simulink model "pendule_simple"  (R2021a)
settings: Solver=VariableStepAuto  StartTime=0.0  StopTime=10.0  RelTol=1e-3
libraries: simulink x1
settings Model: Creator=ialouane  LastModifiedBy=ialouane

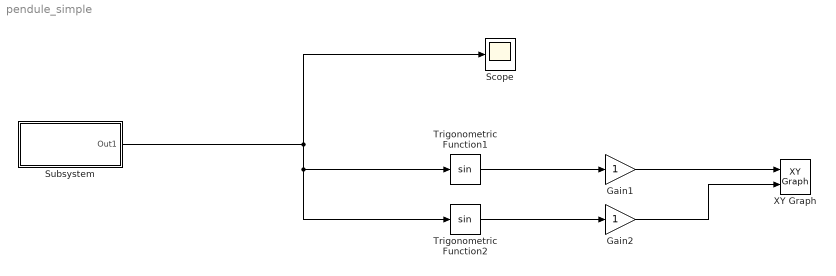
== system pendule_simple ==
  Gain1 : Gain
  Gain2 : Gain
  Scope : Scope
  Subsystem : Subsystem
  Trigonometric Function1 : Trigonometry
  Trigonometric Function2 : Trigonometry
  XY Graph : simulink/Sinks/XY Graph  xmin=-1  xmax=1  ymin=-1  ymax=1  st=-1
  wires:
  Trigonometric Function2/1 -> Gain2/1
  Trigonometric Function1/1 -> Gain1/1
  Gain1/1 -> XY Graph/1
  Gain2/1 -> XY Graph/2
  Subsystem/1(Out1) -> Trigonometric Function2/1, Trigonometric Function1/1, Scope/1

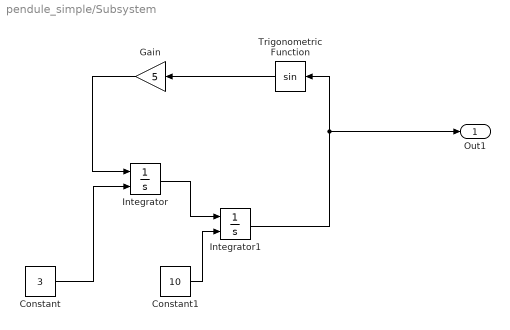
== system pendule_simple/Subsystem ==
  Constant : Constant  Value=3
  Constant1 : Constant  Value=10
  Gain : Gain  Gain=5
  Integrator : Integrator  InitialConditionSource=external
  Integrator1 : Integrator  InitialConditionSource=external
  Trigonometric Function : Trigonometry
  Out1 : Outport
  wires:
  Integrator/1 -> Integrator1/1
  Constant/1 -> Integrator/2
  Trigonometric Function/1 -> Gain/1
  Gain/1 -> Integrator/1
  Integrator1/1 -> Out1/1, Trigonometric Function/1
  Constant1/1 -> Integrator1/2
